simulink model "test_qr4_est"  (Simulink 7.0)
settings: Solver=ode45  StartTime=0.0  StopTime=10.0  RelTol=1e-3
libraries: xbsIndex_r4 x1048
(part 2 of 18)

== system test_qr4_est/r4_dit_fft/r4_dit_stage_2 ==
  a_in : Inport  OutDataType=sfix(16)  OutScaling=2^0
  b_in : Inport  Port=2  OutDataType=sfix(16)  OutScaling=2^0
  c_in : Inport  Port=3  OutDataType=sfix(16)  OutScaling=2^0
  d_in : Inport  Port=4  OutDataType=sfix(16)  OutScaling=2^0
  sync_in : Inport  Port=5  OutDataType=sfix(16)  OutScaling=2^0
  quadplex_commutator : Subsystem  mask(Quadplex Commutator){log4_size=4, n_bits=10, use_bram=off}
      mask prompts: log4_size "Log4 Block Size"; n_bits "Bit Width"; use_bram "Use BRAM"
      mask help: The quadplex commutator performs a "quarter-blockwise" commutation of the four inputs. A "block" is 4^log4_size consecutive samples (i.e. always a power of 4). sync_in precedes the first data input sample by one clock cycle. Overall latency from sync_in to sync_out is 2^(log4_size)+2^(log4_size-1)+2.
      settings: AttributesFormatString=|
      | size = 256
      | 0/4 bram
      mask Help:
      | <pre>
      | Description::
      | 
      | The quadplex commutator performs a "quarter-blockwise" commutation of the four inputs.
      | A "block" is 4^log4_size consecutive samples (i.e. always a power of 4).
      | 
      | sync_in precedes the first data input sample by one clock cycle.
      | sync_out precedes the corresponding output sample by one clock cycle.
      | Overall latency from sync_in to sync_out is 2^(log4_size)+2^(log4_size-1)+2.
      | 
      | Mask Parameters::
      | 
      | Log4 Block Size (log4_size): The base-4 logarithm of the length of one complete input block.
      | This MUST be an integer because the current implementation requires that
      | the input block size MUST be a power of 4.  (aka "N")
      | 
      | Bit Width (n_bits): Specifies the width of the real/imaginary components.
      | Width of each component is assumed equal.
      | 
      | Use BRAM (use_bram): Check this checkbox to implement the internal delays using BRAM.
      | If unchecked, the internal delays will be implemented using SLR16 elements.
      | </pre>
  r4_butterfly : Subsystem  mask(Radix-4 Butterfly){n_bits=10, shift=0, quantization=Truncate, add_latency=1}
      mask prompts: n_bits "Bit Width In"; shift "Shift Bits"; add_latency "Adder Latency"
      mask help: The radix-4 butterfly performs a 4 point FFT on its four inputs (a_in,b_in,c_in,d_in), which are assumed to be in normal order. Its ouputs (a_out,b_out,c_out,d_out) are in bit-reversed order (despite the lexigraphical ordering of the output port names).
      settings: AttributesFormatString=shift 0
      mask Help:
      | <pre>
      | Description::
      | 
      | The radix-4 butterfly performs a 4 point FFT on its four inputs (a_in,b_in,c_in,d_in),
      | which are assumed to be in normal order.  Its ouputs (a_out,b_out,c_out,d_out) are
      | in bit-reversed order (despite the lexigraphical ordering of the output port names).
      | 
      | The outputs are two bits wider than the inputs.
      | The output precision (i.e. the number of fractional bits) stays the same.
      | 
      | Mask Parameters::
      | 
      | Bit Width In (n_bits): Specifies the width of the real/imaginary components.
      | Width of each component is assumed equal.
      | 
      | Shift Bits (shift): Specifies how many bits to shift (down) by.  A positive value causes
      | the specified number of least significant bits to be dropped.  Usually zero or positive values
      | are used to permit or limit bit growth, but negative values can be used to induce bit growth.
      | 
      | Quantization (quantization): Specifies quantization handling (when shift bits > 0).
      | 
      | Adder Latency (add_latency): Latency to use for the underlying real adders.
      | </pre>
      mask StyleString: edit,edit,popup(Truncate|Round  (unbiased: +/- Inf)|Round  (unbiased: Even Values)),edit
  r4_twiddle : Subsystem  mask(Radix-4 General Twiddle Stage){n_stages=5, cur_stage=2, decimation=Time, n_bits=10, bin_pt=7, n_bits_w=9, use_bram=off, mult_latency=3, add_latency=1}
      mask prompts: n_stages "Total Stages"; cur_stage "Current Stage"; decimation "Decimation Mode"; n_bits "Number of Bits In/Out"; bin_pt "Binary Point In/Out"; n_bits_w "Twiddle Coefficient Bitwidth"; use_bram "Use BRAM For Twiddle Coefficients"; mult_latency "Multiplier Latency"; add_latency "Adder Latency"
      mask help: A general twiddle stage for radix-4 Fast Fourier Transforms. Can be used in Decimation in Time (i.e. twiddles before butterflies) or Decimation in Frequency (i.e. twiddles after butterflies) FFTs. Regardless of the decimation mode, the FFT is assumed to have inputs in normal order and outputs in bit-reversed order.
      settings: AttributesFormatString=4 twiddles in dist
      mask Help:
      | <pre>
      | Description::
      | 
      | A general twiddle stage for radix-2 Fast Fourier Transforms.
      | 
      | Can be used in  Decimation in Time (i.e. twiddles before butterflies) or Decimation in Frequency
      | (i.e. twiddles after butterflies) FFTs.  Regardless of the decimation mode, the FFT is assumed
      | to have inputs in normal order and outputs in bit-reversed order.
      | 
      | Input a_in is passed through unchanged to a_out, while inputs b, c, and d are passed through
      | to outputs bw, cw, and dw after being "twiddled".  Since twiddling is effectively multiplication
      | by a complex number with unity magnitude, the bit respresentation of bw/cw/dw is the same
      | as b/c/d (i.e. twiddling does not cause bit growth).  Input a_in is assumed to have the same bit
      | width as b.  Thus, a_in, a_out, b, c, d, bw, cw, and dw all have the same bit representation.
      | 
      | Mask Parameters::
      | 
      | Total Stages (n_stages):  The number of total stages in the FFT.
      | The FFT will have 4^n_stages points.
      | 
      | Current Stage (cur_stage):  The number of the current stage for which this block should
      | generate twiddle coefficients.  Valid values are 2 through n_stages, inclusive.  Note that
      | stages are counted from 1 to n_stages for DIT (i.e. cur_stage==1 for the first stage) and
      | n_stages to 1 for DIF (i.e. cur_stage==1 for the last stage).
      | 
      | Decimation Mode (decimation): The decimation mode of the FFT.
      | 
      | Number of Bits In/Out (n_bits): Specifies the width of the real/imaginary
      | components of ports a_in, b, a_out, bw.  Assumed equal for both components.
      | 
      | Binary Point In/Out (bin_pt): Specifies the binary point position of the real/imaginary
      | components of ports a_in, b, a_out, bw.  Assumed equal for both components.
      | 
      | Twiddle Coefficient Bitwidth (n_bits_w): Specifies the width of the real/imaginary
      | components of the twiddle coefficients.  Assumed equal for both components.
      | 
      | Use BRAM for Twiddle Coefficients (use_bram): Check this checkbox to store twiddle
      | coefficients in BRAM.  If unchecked, the twiddle coefficients will be sored in distributed
      | memory (i.e. slices).
      | 
      | Multiplier Latency (mult_latency): Latency to use for the underlying real multipliers.
      | 
      | Adder Latency (add_latency): Latency to use for the underlying real adders.
      mask StyleString: edit,edit,popup(Time|Frequency),edit,edit,edit,checkbox,edit,edit
  a_out : Outport  OutDataType=sfix(16)  OutScaling=2^0
  b_out : Outport  Port=2  OutDataType=sfix(16)  OutScaling=2^0
  c_out : Outport  Port=3  OutDataType=sfix(16)  OutScaling=2^0
  d_out : Outport  Port=4  OutDataType=sfix(16)  OutScaling=2^0
  sync_out : Outport  Port=5  OutDataType=sfix(16)  OutScaling=2^0
  wires:
  r4_butterfly/5(sync_out) -> sync_out/1
  r4_butterfly/4(d_out) -> d_out/1
  r4_butterfly/3(c_out) -> c_out/1
  r4_butterfly/2(b_out) -> b_out/1
  r4_butterfly/1(a_out) -> a_out/1
  sync_in/1 -> quadplex_commutator/5(sync_in)
  d_in/1 -> quadplex_commutator/4(d)
  c_in/1 -> quadplex_commutator/3(c)
  b_in/1 -> quadplex_commutator/2(b)
  a_in/1 -> quadplex_commutator/1(a)
  r4_twiddle/5(sync_out) -> r4_butterfly/5(sync_in)
  r4_twiddle/4(dw) -> r4_butterfly/4(d_in)
  r4_twiddle/3(cw) -> r4_butterfly/3(c_in)
  r4_twiddle/2(bw) -> r4_butterfly/2(b_in)
  r4_twiddle/1(a_out) -> r4_butterfly/1(a_in)
  quadplex_commutator/5(sync_out) -> r4_twiddle/5(sync_in)
  quadplex_commutator/4(abcd3) -> r4_twiddle/4(d)
  quadplex_commutator/3(abcd2) -> r4_twiddle/3(c)
  quadplex_commutator/2(abcd1) -> r4_twiddle/2(b)
  quadplex_commutator/1(abcd0) -> r4_twiddle/1(a_in)

== system test_qr4_est/r4_dit_fft/r4_dit_stage_3 ==
  a_in : Inport  OutDataType=sfix(16)  OutScaling=2^0
  b_in : Inport  Port=2  OutDataType=sfix(16)  OutScaling=2^0
  c_in : Inport  Port=3  OutDataType=sfix(16)  OutScaling=2^0
  d_in : Inport  Port=4  OutDataType=sfix(16)  OutScaling=2^0
  sync_in : Inport  Port=5  OutDataType=sfix(16)  OutScaling=2^0
  quadplex_commutator : Subsystem  mask(Quadplex Commutator){log4_size=3, n_bits=12, use_bram=off}
      mask prompts: log4_size "Log4 Block Size"; n_bits "Bit Width"; use_bram "Use BRAM"
      mask help: The quadplex commutator performs a "quarter-blockwise" commutation of the four inputs. A "block" is 4^log4_size consecutive samples (i.e. always a power of 4). sync_in precedes the first data input sample by one clock cycle. Overall latency from sync_in to sync_out is 2^(log4_size)+2^(log4_size-1)+2.
      settings: AttributesFormatString=|
      | size = 64
      | 0/4 bram
      mask Help:
      | <pre>
      | Description::
      | 
      | The quadplex commutator performs a "quarter-blockwise" commutation of the four inputs.
      | A "block" is 4^log4_size consecutive samples (i.e. always a power of 4).
      | 
      | sync_in precedes the first data input sample by one clock cycle.
      | sync_out precedes the corresponding output sample by one clock cycle.
      | Overall latency from sync_in to sync_out is 2^(log4_size)+2^(log4_size-1)+2.
      | 
      | Mask Parameters::
      | 
      | Log4 Block Size (log4_size): The base-4 logarithm of the length of one complete input block.
      | This MUST be an integer because the current implementation requires that
      | the input block size MUST be a power of 4.  (aka "N")
      | 
      | Bit Width (n_bits): Specifies the width of the real/imaginary components.
      | Width of each component is assumed equal.
      | 
      | Use BRAM (use_bram): Check this checkbox to implement the internal delays using BRAM.
      | If unchecked, the internal delays will be implemented using SLR16 elements.
      | </pre>
  r4_butterfly : Subsystem  mask(Radix-4 Butterfly){n_bits=12, shift=0, quantization=Truncate, add_latency=1}
      mask prompts: n_bits "Bit Width In"; shift "Shift Bits"; add_latency "Adder Latency"
      mask help: The radix-4 butterfly performs a 4 point FFT on its four inputs (a_in,b_in,c_in,d_in), which are assumed to be in normal order. Its ouputs (a_out,b_out,c_out,d_out) are in bit-reversed order (despite the lexigraphical ordering of the output port names).
      settings: AttributesFormatString=shift 0
      mask Help:
      | <pre>
      | Description::
      | 
      | The radix-4 butterfly performs a 4 point FFT on its four inputs (a_in,b_in,c_in,d_in),
      | which are assumed to be in normal order.  Its ouputs (a_out,b_out,c_out,d_out) are
      | in bit-reversed order (despite the lexigraphical ordering of the output port names).
      | 
      | The outputs are two bits wider than the inputs.
      | The output precision (i.e. the number of fractional bits) stays the same.
      | 
      | Mask Parameters::
      | 
      | Bit Width In (n_bits): Specifies the width of the real/imaginary components.
      | Width of each component is assumed equal.
      | 
      | Shift Bits (shift): Specifies how many bits to shift (down) by.  A positive value causes
      | the specified number of least significant bits to be dropped.  Usually zero or positive values
      | are used to permit or limit bit growth, but negative values can be used to induce bit growth.
      | 
      | Quantization (quantization): Specifies quantization handling (when shift bits > 0).
      | 
      | Adder Latency (add_latency): Latency to use for the underlying real adders.
      | </pre>
      mask StyleString: edit,edit,popup(Truncate|Round  (unbiased: +/- Inf)|Round  (unbiased: Even Values)),edit
  r4_twiddle : Subsystem  mask(Radix-4 General Twiddle Stage){n_stages=5, cur_stage=3, decimation=Time, n_bits=12, bin_pt=7, n_bits_w=9, use_bram=off, mult_latency=3, add_latency=1}
      mask prompts: n_stages "Total Stages"; cur_stage "Current Stage"; decimation "Decimation Mode"; n_bits "Number of Bits In/Out"; bin_pt "Binary Point In/Out"; n_bits_w "Twiddle Coefficient Bitwidth"; use_bram "Use BRAM For Twiddle Coefficients"; mult_latency "Multiplier Latency"; add_latency "Adder Latency"
      mask help: A general twiddle stage for radix-4 Fast Fourier Transforms. Can be used in Decimation in Time (i.e. twiddles before butterflies) or Decimation in Frequency (i.e. twiddles after butterflies) FFTs. Regardless of the decimation mode, the FFT is assumed to have inputs in normal order and outputs in bit-reversed order.
      settings: AttributesFormatString=16 twiddles in dist
      mask Help:
      | <pre>
      | Description::
      | 
      | A general twiddle stage for radix-2 Fast Fourier Transforms.
      | 
      | Can be used in  Decimation in Time (i.e. twiddles before butterflies) or Decimation in Frequency
      | (i.e. twiddles after butterflies) FFTs.  Regardless of the decimation mode, the FFT is assumed
      | to have inputs in normal order and outputs in bit-reversed order.
      | 
      | Input a_in is passed through unchanged to a_out, while inputs b, c, and d are passed through
      | to outputs bw, cw, and dw after being "twiddled".  Since twiddling is effectively multiplication
      | by a complex number with unity magnitude, the bit respresentation of bw/cw/dw is the same
      | as b/c/d (i.e. twiddling does not cause bit growth).  Input a_in is assumed to have the same bit
      | width as b.  Thus, a_in, a_out, b, c, d, bw, cw, and dw all have the same bit representation.
      | 
      | Mask Parameters::
      | 
      | Total Stages (n_stages):  The number of total stages in the FFT.
      | The FFT will have 4^n_stages points.
      | 
      | Current Stage (cur_stage):  The number of the current stage for which this block should
      | generate twiddle coefficients.  Valid values are 2 through n_stages, inclusive.  Note that
      | stages are counted from 1 to n_stages for DIT (i.e. cur_stage==1 for the first stage) and
      | n_stages to 1 for DIF (i.e. cur_stage==1 for the last stage).
      | 
      | Decimation Mode (decimation): The decimation mode of the FFT.
      | 
      | Number of Bits In/Out (n_bits): Specifies the width of the real/imaginary
      | components of ports a_in, b, a_out, bw.  Assumed equal for both components.
      | 
      | Binary Point In/Out (bin_pt): Specifies the binary point position of the real/imaginary
      | components of ports a_in, b, a_out, bw.  Assumed equal for both components.
      | 
      | Twiddle Coefficient Bitwidth (n_bits_w): Specifies the width of the real/imaginary
      | components of the twiddle coefficients.  Assumed equal for both components.
      | 
      | Use BRAM for Twiddle Coefficients (use_bram): Check this checkbox to store twiddle
      | coefficients in BRAM.  If unchecked, the twiddle coefficients will be sored in distributed
      | memory (i.e. slices).
      | 
      | Multiplier Latency (mult_latency): Latency to use for the underlying real multipliers.
      | 
      | Adder Latency (add_latency): Latency to use for the underlying real adders.
      mask StyleString: edit,edit,popup(Time|Frequency),edit,edit,edit,checkbox,edit,edit
  a_out : Outport  OutDataType=sfix(16)  OutScaling=2^0
  b_out : Outport  Port=2  OutDataType=sfix(16)  OutScaling=2^0
  c_out : Outport  Port=3  OutDataType=sfix(16)  OutScaling=2^0
  d_out : Outport  Port=4  OutDataType=sfix(16)  OutScaling=2^0
  sync_out : Outport  Port=5  OutDataType=sfix(16)  OutScaling=2^0
  wires:
  r4_butterfly/5(sync_out) -> sync_out/1
  r4_butterfly/4(d_out) -> d_out/1
  r4_butterfly/3(c_out) -> c_out/1
  r4_butterfly/2(b_out) -> b_out/1
  r4_butterfly/1(a_out) -> a_out/1
  sync_in/1 -> quadplex_commutator/5(sync_in)
  d_in/1 -> quadplex_commutator/4(d)
  c_in/1 -> quadplex_commutator/3(c)
  b_in/1 -> quadplex_commutator/2(b)
  a_in/1 -> quadplex_commutator/1(a)
  r4_twiddle/5(sync_out) -> r4_butterfly/5(sync_in)
  r4_twiddle/4(dw) -> r4_butterfly/4(d_in)
  r4_twiddle/3(cw) -> r4_butterfly/3(c_in)
  r4_twiddle/2(bw) -> r4_butterfly/2(b_in)
  r4_twiddle/1(a_out) -> r4_butterfly/1(a_in)
  quadplex_commutator/5(sync_out) -> r4_twiddle/5(sync_in)
  quadplex_commutator/4(abcd3) -> r4_twiddle/4(d)
  quadplex_commutator/3(abcd2) -> r4_twiddle/3(c)
  quadplex_commutator/2(abcd1) -> r4_twiddle/2(b)
  quadplex_commutator/1(abcd0) -> r4_twiddle/1(a_in)

== system test_qr4_est/r4_dit_fft/r4_dit_stage_4 ==
  a_in : Inport  OutDataType=sfix(16)  OutScaling=2^0
  b_in : Inport  Port=2  OutDataType=sfix(16)  OutScaling=2^0
  c_in : Inport  Port=3  OutDataType=sfix(16)  OutScaling=2^0
  d_in : Inport  Port=4  OutDataType=sfix(16)  OutScaling=2^0
  sync_in : Inport  Port=5  OutDataType=sfix(16)  OutScaling=2^0
  quadplex_commutator : Subsystem  mask(Quadplex Commutator){log4_size=2, n_bits=14, use_bram=off}
      mask prompts: log4_size "Log4 Block Size"; n_bits "Bit Width"; use_bram "Use BRAM"
      mask help: The quadplex commutator performs a "quarter-blockwise" commutation of the four inputs. A "block" is 4^log4_size consecutive samples (i.e. always a power of 4). sync_in precedes the first data input sample by one clock cycle. Overall latency from sync_in to sync_out is 2^(log4_size)+2^(log4_size-1)+2.
      settings: AttributesFormatString=|
      | size = 16
      | 0/4 bram
      mask Help:
      | <pre>
      | Description::
      | 
      | The quadplex commutator performs a "quarter-blockwise" commutation of the four inputs.
      | A "block" is 4^log4_size consecutive samples (i.e. always a power of 4).
      | 
      | sync_in precedes the first data input sample by one clock cycle.
      | sync_out precedes the corresponding output sample by one clock cycle.
      | Overall latency from sync_in to sync_out is 2^(log4_size)+2^(log4_size-1)+2.
      | 
      | Mask Parameters::
      | 
      | Log4 Block Size (log4_size): The base-4 logarithm of the length of one complete input block.
      | This MUST be an integer because the current implementation requires that
      | the input block size MUST be a power of 4.  (aka "N")
      | 
      | Bit Width (n_bits): Specifies the width of the real/imaginary components.
      | Width of each component is assumed equal.
      | 
      | Use BRAM (use_bram): Check this checkbox to implement the internal delays using BRAM.
      | If unchecked, the internal delays will be implemented using SLR16 elements.
      | </pre>
  r4_butterfly : Subsystem  mask(Radix-4 Butterfly){n_bits=14, shift=0, quantization=Truncate, add_latency=1}
      mask prompts: n_bits "Bit Width In"; shift "Shift Bits"; add_latency "Adder Latency"
      mask help: The radix-4 butterfly performs a 4 point FFT on its four inputs (a_in,b_in,c_in,d_in), which are assumed to be in normal order. Its ouputs (a_out,b_out,c_out,d_out) are in bit-reversed order (despite the lexigraphical ordering of the output port names).
      settings: AttributesFormatString=shift 0
      mask Help:
      | <pre>
      | Description::
      | 
      | The radix-4 butterfly performs a 4 point FFT on its four inputs (a_in,b_in,c_in,d_in),
      | which are assumed to be in normal order.  Its ouputs (a_out,b_out,c_out,d_out) are
      | in bit-reversed order (despite the lexigraphical ordering of the output port names).
      | 
      | The outputs are two bits wider than the inputs.
      | The output precision (i.e. the number of fractional bits) stays the same.
      | 
      | Mask Parameters::
      | 
      | Bit Width In (n_bits): Specifies the width of the real/imaginary components.
      | Width of each component is assumed equal.
      | 
      | Shift Bits (shift): Specifies how many bits to shift (down) by.  A positive value causes
      | the specified number of least significant bits to be dropped.  Usually zero or positive values
      | are used to permit or limit bit growth, but negative values can be used to induce bit growth.
      | 
      | Quantization (quantization): Specifies quantization handling (when shift bits > 0).
      | 
      | Adder Latency (add_latency): Latency to use for the underlying real adders.
      | </pre>
      mask StyleString: edit,edit,popup(Truncate|Round  (unbiased: +/- Inf)|Round  (unbiased: Even Values)),edit
  r4_twiddle : Subsystem  mask(Radix-4 General Twiddle Stage){n_stages=5, cur_stage=4, decimation=Time, n_bits=14, bin_pt=7, n_bits_w=9, use_bram=off, mult_latency=3, add_latency=1}
      mask prompts: n_stages "Total Stages"; cur_stage "Current Stage"; decimation "Decimation Mode"; n_bits "Number of Bits In/Out"; bin_pt "Binary Point In/Out"; n_bits_w "Twiddle Coefficient Bitwidth"; use_bram "Use BRAM For Twiddle Coefficients"; mult_latency "Multiplier Latency"; add_latency "Adder Latency"
      mask help: A general twiddle stage for radix-4 Fast Fourier Transforms. Can be used in Decimation in Time (i.e. twiddles before butterflies) or Decimation in Frequency (i.e. twiddles after butterflies) FFTs. Regardless of the decimation mode, the FFT is assumed to have inputs in normal order and outputs in bit-reversed order.
      settings: AttributesFormatString=64 twiddles in dist
      mask Help:
      | <pre>
      | Description::
      | 
      | A general twiddle stage for radix-2 Fast Fourier Transforms.
      | 
      | Can be used in  Decimation in Time (i.e. twiddles before butterflies) or Decimation in Frequency
      | (i.e. twiddles after butterflies) FFTs.  Regardless of the decimation mode, the FFT is assumed
      | to have inputs in normal order and outputs in bit-reversed order.
      | 
      | Input a_in is passed through unchanged to a_out, while inputs b, c, and d are passed through
      | to outputs bw, cw, and dw after being "twiddled".  Since twiddling is effectively multiplication
      | by a complex number with unity magnitude, the bit respresentation of bw/cw/dw is the same
      | as b/c/d (i.e. twiddling does not cause bit growth).  Input a_in is assumed to have the same bit
      | width as b.  Thus, a_in, a_out, b, c, d, bw, cw, and dw all have the same bit representation.
      | 
      | Mask Parameters::
      | 
      | Total Stages (n_stages):  The number of total stages in the FFT.
      | The FFT will have 4^n_stages points.
      | 
      | Current Stage (cur_stage):  The number of the current stage for which this block should
      | generate twiddle coefficients.  Valid values are 2 through n_stages, inclusive.  Note that
      | stages are counted from 1 to n_stages for DIT (i.e. cur_stage==1 for the first stage) and
      | n_stages to 1 for DIF (i.e. cur_stage==1 for the last stage).
      | 
      | Decimation Mode (decimation): The decimation mode of the FFT.
      | 
      | Number of Bits In/Out (n_bits): Specifies the width of the real/imaginary
      | components of ports a_in, b, a_out, bw.  Assumed equal for both components.
      | 
      | Binary Point In/Out (bin_pt): Specifies the binary point position of the real/imaginary
      | components of ports a_in, b, a_out, bw.  Assumed equal for both components.
      | 
      | Twiddle Coefficient Bitwidth (n_bits_w): Specifies the width of the real/imaginary
      | components of the twiddle coefficients.  Assumed equal for both components.
      | 
      | Use BRAM for Twiddle Coefficients (use_bram): Check this checkbox to store twiddle
      | coefficients in BRAM.  If unchecked, the twiddle coefficients will be sored in distributed
      | memory (i.e. slices).
      | 
      | Multiplier Latency (mult_latency): Latency to use for the underlying real multipliers.
      | 
      | Adder Latency (add_latency): Latency to use for the underlying real adders.
      mask StyleString: edit,edit,popup(Time|Frequency),edit,edit,edit,checkbox,edit,edit
  a_out : Outport  OutDataType=sfix(16)  OutScaling=2^0
  b_out : Outport  Port=2  OutDataType=sfix(16)  OutScaling=2^0
  c_out : Outport  Port=3  OutDataType=sfix(16)  OutScaling=2^0
  d_out : Outport  Port=4  OutDataType=sfix(16)  OutScaling=2^0
  sync_out : Outport  Port=5  OutDataType=sfix(16)  OutScaling=2^0
  wires:
  r4_butterfly/5(sync_out) -> sync_out/1
  r4_butterfly/4(d_out) -> d_out/1
  r4_butterfly/3(c_out) -> c_out/1
  r4_butterfly/2(b_out) -> b_out/1
  r4_butterfly/1(a_out) -> a_out/1
  sync_in/1 -> quadplex_commutator/5(sync_in)
  d_in/1 -> quadplex_commutator/4(d)
  c_in/1 -> quadplex_commutator/3(c)
  b_in/1 -> quadplex_commutator/2(b)
  a_in/1 -> quadplex_commutator/1(a)
  r4_twiddle/5(sync_out) -> r4_butterfly/5(sync_in)
  r4_twiddle/4(dw) -> r4_butterfly/4(d_in)
  r4_twiddle/3(cw) -> r4_butterfly/3(c_in)
  r4_twiddle/2(bw) -> r4_butterfly/2(b_in)
  r4_twiddle/1(a_out) -> r4_butterfly/1(a_in)
  quadplex_commutator/5(sync_out) -> r4_twiddle/5(sync_in)
  quadplex_commutator/4(abcd3) -> r4_twiddle/4(d)
  quadplex_commutator/3(abcd2) -> r4_twiddle/3(c)
  quadplex_commutator/2(abcd1) -> r4_twiddle/2(b)
  quadplex_commutator/1(abcd0) -> r4_twiddle/1(a_in)

== system test_qr4_est/r4_dit_fft/r4_dit_stage_5 ==
  a_in : Inport  OutDataType=sfix(16)  OutScaling=2^0
  b_in : Inport  Port=2  OutDataType=sfix(16)  OutScaling=2^0
  c_in : Inport  Port=3  OutDataType=sfix(16)  OutScaling=2^0
  d_in : Inport  Port=4  OutDataType=sfix(16)  OutScaling=2^0
  sync_in : Inport  Port=5  OutDataType=sfix(16)  OutScaling=2^0
  quadplex_commutator : Subsystem  mask(Quadplex Commutator){log4_size=1, n_bits=16, use_bram=off}
      mask prompts: log4_size "Log4 Block Size"; n_bits "Bit Width"; use_bram "Use BRAM"
      mask help: The quadplex commutator performs a "quarter-blockwise" commutation of the four inputs. A "block" is 4^log4_size consecutive samples (i.e. always a power of 4). sync_in precedes the first data input sample by one clock cycle. Overall latency from sync_in to sync_out is 2^(log4_size)+2^(log4_size-1)+2.
      settings: AttributesFormatString=|
      | size = 4
      | 0/4 bram
      mask Help:
      | <pre>
      | Description::
      | 
      | The quadplex commutator performs a "quarter-blockwise" commutation of the four inputs.
      | A "block" is 4^log4_size consecutive samples (i.e. always a power of 4).
      | 
      | sync_in precedes the first data input sample by one clock cycle.
      | sync_out precedes the corresponding output sample by one clock cycle.
      | Overall latency from sync_in to sync_out is 2^(log4_size)+2^(log4_size-1)+2.
      | 
      | Mask Parameters::
      | 
      | Log4 Block Size (log4_size): The base-4 logarithm of the length of one complete input block.
      | This MUST be an integer because the current implementation requires that
      | the input block size MUST be a power of 4.  (aka "N")
      | 
      | Bit Width (n_bits): Specifies the width of the real/imaginary components.
      | Width of each component is assumed equal.
      | 
      | Use BRAM (use_bram): Check this checkbox to implement the internal delays using BRAM.
      | If unchecked, the internal delays will be implemented using SLR16 elements.
      | </pre>
  r4_butterfly : Subsystem  mask(Radix-4 Butterfly){n_bits=16, shift=0, quantization=Truncate, add_latency=1}
      mask prompts: n_bits "Bit Width In"; shift "Shift Bits"; add_latency "Adder Latency"
      mask help: The radix-4 butterfly performs a 4 point FFT on its four inputs (a_in,b_in,c_in,d_in), which are assumed to be in normal order. Its ouputs (a_out,b_out,c_out,d_out) are in bit-reversed order (despite the lexigraphical ordering of the output port names).
      settings: AttributesFormatString=shift 0
      mask Help:
      | <pre>
      | Description::
      | 
      | The radix-4 butterfly performs a 4 point FFT on its four inputs (a_in,b_in,c_in,d_in),
      | which are assumed to be in normal order.  Its ouputs (a_out,b_out,c_out,d_out) are
      | in bit-reversed order (despite the lexigraphical ordering of the output port names).
      | 
      | The outputs are two bits wider than the inputs.
      | The output precision (i.e. the number of fractional bits) stays the same.
      | 
      | Mask Parameters::
      | 
      | Bit Width In (n_bits): Specifies the width of the real/imaginary components.
      | Width of each component is assumed equal.
      | 
      | Shift Bits (shift): Specifies how many bits to shift (down) by.  A positive value causes
      | the specified number of least significant bits to be dropped.  Usually zero or positive values
      | are used to permit or limit bit growth, but negative values can be used to induce bit growth.
      | 
      | Quantization (quantization): Specifies quantization handling (when shift bits > 0).
      | 
      | Adder Latency (add_latency): Latency to use for the underlying real adders.
      | </pre>
      mask StyleString: edit,edit,popup(Truncate|Round  (unbiased: +/- Inf)|Round  (unbiased: Even Values)),edit
  r4_twiddle : Subsystem  mask(Radix-4 General Twiddle Stage){n_stages=5, cur_stage=5, decimation=Time, n_bits=16, bin_pt=7, n_bits_w=9, use_bram=on, mult_latency=3, add_latency=1}
      mask prompts: n_stages "Total Stages"; cur_stage "Current Stage"; decimation "Decimation Mode"; n_bits "Number of Bits In/Out"; bin_pt "Binary Point In/Out"; n_bits_w "Twiddle Coefficient Bitwidth"; use_bram "Use BRAM For Twiddle Coefficients"; mult_latency "Multiplier Latency"; add_latency "Adder Latency"
      mask help: A general twiddle stage for radix-4 Fast Fourier Transforms. Can be used in Decimation in Time (i.e. twiddles before butterflies) or Decimation in Frequency (i.e. twiddles after butterflies) FFTs. Regardless of the decimation mode, the FFT is assumed to have inputs in normal order and outputs in bit-reversed order.
      settings: AttributesFormatString=256 twiddles in bram
      mask Help:
      | <pre>
      | Description::
      | 
      | A general twiddle stage for radix-2 Fast Fourier Transforms.
      | 
      | Can be used in  Decimation in Time (i.e. twiddles before butterflies) or Decimation in Frequency
      | (i.e. twiddles after butterflies) FFTs.  Regardless of the decimation mode, the FFT is assumed
      | to have inputs in normal order and outputs in bit-reversed order.
      | 
      | Input a_in is passed through unchanged to a_out, while inputs b, c, and d are passed through
      | to outputs bw, cw, and dw after being "twiddled".  Since twiddling is effectively multiplication
      | by a complex number with unity magnitude, the bit respresentation of bw/cw/dw is the same
      | as b/c/d (i.e. twiddling does not cause bit growth).  Input a_in is assumed to have the same bit
      | width as b.  Thus, a_in, a_out, b, c, d, bw, cw, and dw all have the same bit representation.
      | 
      | Mask Parameters::
      | 
      | Total Stages (n_stages):  The number of total stages in the FFT.
      | The FFT will have 4^n_stages points.
      | 
      | Current Stage (cur_stage):  The number of the current stage for which this block should
      | generate twiddle coefficients.  Valid values are 2 through n_stages, inclusive.  Note that
      | stages are counted from 1 to n_stages for DIT (i.e. cur_stage==1 for the first stage) and
      | n_stages to 1 for DIF (i.e. cur_stage==1 for the last stage).
      | 
      | Decimation Mode (decimation): The decimation mode of the FFT.
      | 
      | Number of Bits In/Out (n_bits): Specifies the width of the real/imaginary
      | components of ports a_in, b, a_out, bw.  Assumed equal for both components.
      | 
      | Binary Point In/Out (bin_pt): Specifies the binary point position of the real/imaginary
      | components of ports a_in, b, a_out, bw.  Assumed equal for both components.
      | 
      | Twiddle Coefficient Bitwidth (n_bits_w): Specifies the width of the real/imaginary
      | components of the twiddle coefficients.  Assumed equal for both components.
      | 
      | Use BRAM for Twiddle Coefficients (use_bram): Check this checkbox to store twiddle
      | coefficients in BRAM.  If unchecked, the twiddle coefficients will be sored in distributed
      | memory (i.e. slices).
      | 
      | Multiplier Latency (mult_latency): Latency to use for the underlying real multipliers.
      | 
      | Adder Latency (add_latency): Latency to use for the underlying real adders.
      mask StyleString: edit,edit,popup(Time|Frequency),edit,edit,edit,checkbox,edit,edit
  a_out : Outport  OutDataType=sfix(16)  OutScaling=2^0
  b_out : Outport  Port=2  OutDataType=sfix(16)  OutScaling=2^0
  c_out : Outport  Port=3  OutDataType=sfix(16)  OutScaling=2^0
  d_out : Outport  Port=4  OutDataType=sfix(16)  OutScaling=2^0
  sync_out : Outport  Port=5  OutDataType=sfix(16)  OutScaling=2^0
  wires:
  r4_butterfly/5(sync_out) -> sync_out/1
  r4_butterfly/4(d_out) -> d_out/1
  r4_butterfly/3(c_out) -> c_out/1
  r4_butterfly/2(b_out) -> b_out/1
  r4_butterfly/1(a_out) -> a_out/1
  sync_in/1 -> quadplex_commutator/5(sync_in)
  d_in/1 -> quadplex_commutator/4(d)
  c_in/1 -> quadplex_commutator/3(c)
  b_in/1 -> quadplex_commutator/2(b)
  a_in/1 -> quadplex_commutator/1(a)
  r4_twiddle/5(sync_out) -> r4_butterfly/5(sync_in)
  r4_twiddle/4(dw) -> r4_butterfly/4(d_in)
  r4_twiddle/3(cw) -> r4_butterfly/3(c_in)
  r4_twiddle/2(bw) -> r4_butterfly/2(b_in)
  r4_twiddle/1(a_out) -> r4_butterfly/1(a_in)
  quadplex_commutator/5(sync_out) -> r4_twiddle/5(sync_in)
  quadplex_commutator/4(abcd3) -> r4_twiddle/4(d)
  quadplex_commutator/3(abcd2) -> r4_twiddle/3(c)
  quadplex_commutator/2(abcd1) -> r4_twiddle/2(b)
  quadplex_commutator/1(abcd0) -> r4_twiddle/1(a_in)

== system test_qr4_est/r4_dit_fft/r4_dit_stage_1/quadplex_commutator ==
  a : Inport  OutDataType=sfix(16)  OutScaling=2^0
  b : Inport  Port=2  OutDataType=sfix(16)  OutScaling=2^0
  c : Inport  Port=3  OutDataType=sfix(16)  OutScaling=2^0
  d : Inport  Port=4  OutDataType=sfix(16)  OutScaling=2^0
  sync_in : Inport  Port=5  OutDataType=sfix(16)  OutScaling=2^0
  Terminator : Terminator
  biplex_commutator_01 : Subsystem  mask(Biplex Commutator){log2_size=9, n_bits=8, use_bram=on}
      mask prompts: log2_size "Log2 Block Size"; n_bits "Bit Width"; use_bram "Use BRAM"
      mask help: The biplex commutator commutes the first half of the BloBhi input "block" with the last half of the AloAhi input "block". A "block" is 2^log2_size consecutive samples (i.e. always a power of 2). sync_in precedes the first data input sample by one clock cycle. Overall latency from sync_in to sync_out is 2^(log2_size-1)+1.
      settings: AttributesFormatString=|
      | size = 512
      | delay bram
      mask Help:
      | <pre>
      | Description::
      | 
      | The biplex commutator commutes the first half of the BloBhi input "block"  with the last half
      | of the AloAhi input "block".  A "block" is 2^log2_size consecutive samples (i.e. always a
      | power of 2).
      | 
      | sync_in precedes the first data input sample by one clock cycle.
      | sync_out precedes the corresponding output sample by one clock cycle.
      | Overall latency from sync_in to sync_out is 2^(N-1)+1.
      | 
      | Mask Parameters::
      | 
      | Log 2 Block Size (log2_size): The base-2 logarithm of the length of one complete input block.
      | This MUST be an integer because the current implementation requires that
      | the input block size MUST be a power of 2.  (aka "N")
      | 
      | Bit Width (n_bits): Specifies the width of the real/imaginary components.
      | Width of each component is assumed equal.
      | 
      | Use BRAM (use_bram): Check this checkbox to implement the internal delays using BRAM.
      | If unchecked, the internal delays will be implemented using SLR16 elements.
      | </pre>
  biplex_commutator_23 : Subsystem  mask(Biplex Commutator){log2_size=9, n_bits=8, use_bram=on}
      mask prompts: log2_size "Log2 Block Size"; n_bits "Bit Width"; use_bram "Use BRAM"
      mask help: The biplex commutator commutes the first half of the BloBhi input "block" with the last half of the AloAhi input "block". A "block" is 2^log2_size consecutive samples (i.e. always a power of 2). sync_in precedes the first data input sample by one clock cycle. Overall latency from sync_in to sync_out is 2^(log2_size-1)+1.
      settings: AttributesFormatString=|
      | size = 512
      | delay bram
      mask Help:
      | <pre>
      | Description::
      | 
      | The biplex commutator commutes the first half of the BloBhi input "block"  with the last half
      | of the AloAhi input "block".  A "block" is 2^log2_size consecutive samples (i.e. always a
      | power of 2).
      | 
      | sync_in precedes the first data input sample by one clock cycle.
      | sync_out precedes the corresponding output sample by one clock cycle.
      | Overall latency from sync_in to sync_out is 2^(N-1)+1.
      | 
      | Mask Parameters::
      | 
      | Log 2 Block Size (log2_size): The base-2 logarithm of the length of one complete input block.
      | This MUST be an integer because the current implementation requires that
      | the input block size MUST be a power of 2.  (aka "N")
      | 
      | Bit Width (n_bits): Specifies the width of the real/imaginary components.
      | Width of each component is assumed equal.
      | 
      | Use BRAM (use_bram): Check this checkbox to implement the internal delays using BRAM.
      | If unchecked, the internal delays will be implemented using SLR16 elements.
      | </pre>
  biplex_commutator_ac : Subsystem  mask(Biplex Commutator){log2_size=10, n_bits=8, use_bram=on}
      mask prompts: log2_size "Log2 Block Size"; n_bits "Bit Width"; use_bram "Use BRAM"
      mask help: The biplex commutator commutes the first half of the BloBhi input "block" with the last half of the AloAhi input "block". A "block" is 2^log2_size consecutive samples (i.e. always a power of 2). sync_in precedes the first data input sample by one clock cycle. Overall latency from sync_in to sync_out is 2^(log2_size-1)+1.
      settings: AttributesFormatString=|
      | size = 1024
      | delay bram
      mask Help:
      | <pre>
      | Description::
      | 
      | The biplex commutator commutes the first half of the BloBhi input "block"  with the last half
      | of the AloAhi input "block".  A "block" is 2^log2_size consecutive samples (i.e. always a
      | power of 2).
      | 
      | sync_in precedes the first data input sample by one clock cycle.
      | sync_out precedes the corresponding output sample by one clock cycle.
      | Overall latency from sync_in to sync_out is 2^(N-1)+1.
      | 
      | Mask Parameters::
      | 
      | Log 2 Block Size (log2_size): The base-2 logarithm of the length of one complete input block.
      | This MUST be an integer because the current implementation requires that
      | the input block size MUST be a power of 2.  (aka "N")
      | 
      | Bit Width (n_bits): Specifies the width of the real/imaginary components.
      | Width of each component is assumed equal.
      | 
      | Use BRAM (use_bram): Check this checkbox to implement the internal delays using BRAM.
      | If unchecked, the internal delays will be implemented using SLR16 elements.
      | </pre>
  biplex_commutator_bd : Subsystem  mask(Biplex Commutator){log2_size=10, n_bits=8, use_bram=on}
      mask prompts: log2_size "Log2 Block Size"; n_bits "Bit Width"; use_bram "Use BRAM"
      mask help: The biplex commutator commutes the first half of the BloBhi input "block" with the last half of the AloAhi input "block". A "block" is 2^log2_size consecutive samples (i.e. always a power of 2). sync_in precedes the first data input sample by one clock cycle. Overall latency from sync_in to sync_out is 2^(log2_size-1)+1.
      settings: AttributesFormatString=|
      | size = 1024
      | delay bram
      mask Help:
      | <pre>
      | Description::
      | 
      | The biplex commutator commutes the first half of the BloBhi input "block"  with the last half
      | of the AloAhi input "block".  A "block" is 2^log2_size consecutive samples (i.e. always a
      | power of 2).
      | 
      | sync_in precedes the first data input sample by one clock cycle.
      | sync_out precedes the corresponding output sample by one clock cycle.
      | Overall latency from sync_in to sync_out is 2^(N-1)+1.
      | 
      | Mask Parameters::
      | 
      | Log 2 Block Size (log2_size): The base-2 logarithm of the length of one complete input block.
      | This MUST be an integer because the current implementation requires that
      | the input block size MUST be a power of 2.  (aka "N")
      | 
      | Bit Width (n_bits): Specifies the width of the real/imaginary components.
      | Width of each component is assumed equal.
      | 
      | Use BRAM (use_bram): Check this checkbox to implement the internal delays using BRAM.
      | If unchecked, the internal delays will be implemented using SLR16 elements.
      | </pre>
  abcd0 : Outport  OutDataType=sfix(16)  OutScaling=2^0
  abcd1 : Outport  Port=2  OutDataType=sfix(16)  OutScaling=2^0
  abcd2 : Outport  Port=3  OutDataType=sfix(16)  OutScaling=2^0
  abcd3 : Outport  Port=4  OutDataType=sfix(16)  OutScaling=2^0
  sync_out : Outport  Port=5  OutDataType=sfix(16)  OutScaling=2^0
  wires:
  biplex_commutator_01/3(sync_out) -> Terminator/1
  biplex_commutator_23/3(sync_out) -> sync_out/1
  sync_in/1 -> biplex_commutator_bd/3(sync_in), biplex_commutator_ac/3(sync_in)
  d/1 -> biplex_commutator_bd/2(BloBhi)
  b/1 -> biplex_commutator_bd/1(AloAhi)
  c/1 -> biplex_commutator_ac/2(BloBhi)
  biplex_commutator_bd/3(sync_out) -> biplex_commutator_23/3(sync_in)
  biplex_commutator_bd/2(AhiBhi) -> biplex_commutator_23/2(BloBhi)
  biplex_commutator_ac/3(sync_out) -> biplex_commutator_01/3(sync_in)
  biplex_commutator_bd/1(AloBlo) -> biplex_commutator_01/2(BloBhi)
  biplex_commutator_ac/2(AhiBhi) -> biplex_commutator_23/1(AloAhi)
  biplex_commutator_23/2(AhiBhi) -> abcd3/1
  biplex_commutator_23/1(AloBlo) -> abcd2/1
  biplex_commutator_01/2(AhiBhi) -> abcd1/1
  biplex_commutator_01/1(AloBlo) -> abcd0/1
  a/1 -> biplex_commutator_ac/1(AloAhi)
  biplex_commutator_ac/1(AloBlo) -> biplex_commutator_01/1(AloAhi)
